simulink model "robust_simu"  (R2022a)
settings: Solver=VariableStepAuto  StartTime=0.0  StopTime=600  RelTol=1e-3
values from neighbouring files (symbols this model uses):
  ctrK_A = K.A    [robust.m]
  ctrK_B = K.B    [robust.m]
  ctrK_C = K.C    [robust.m]
  ctrK_D = K.D    [robust.m]
  ctrKpre_A = K_pre.A    [robust.m]
  ctrKpre_B = K_pre.B    [robust.m]
  ctrKpre_C = K_pre.C    [robust.m]
  ctrKpre_D = K_pre.D    [robust.m]
  G_A = sys_G.A    [robust.m]
  G_B = sys_G.B    [robust.m]
  G_C = sys_G.C    [robust.m]
  G_D = sys_G.D    [robust.m]
  Gd_A = sys_Gd.A    [robust.m]
  Gd_B = sys_Gd.B    [robust.m]
  Gd_C = sys_Gd.C    [robust.m]
  Gd_D = sys_Gd.D    [robust.m]
settings Model: Creator=Linxi Ren  LastModifiedBy=Linxi Ren

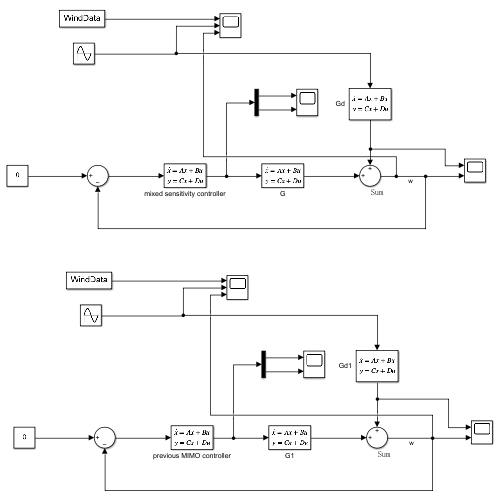
[thumbnail: Simulink's stored preview of the top-level diagram]
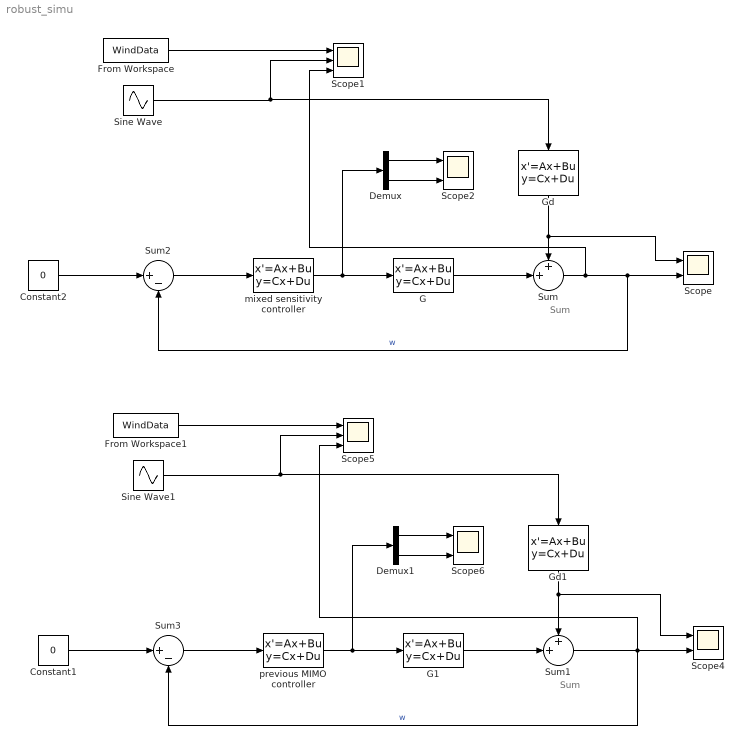
== system robust_simu ==
  note: Sum
  note: Sum
  Constant1 : Constant  Value=0
  Constant2 : Constant  Value=0
  Demux : Demux  Outputs=2
  Demux1 : Demux  Outputs=2
  From Workspace : FromWorkspace  VariableName=WindData  SampleTime=0.01
  From Workspace1 : FromWorkspace  VariableName=WindData  SampleTime=0.01
  G : StateSpace  A=G_A  B=G_B  C=G_C  D=G_D  InitialCondition=0
  G1 : StateSpace  A=G_A  B=G_B  C=G_C  D=G_D  InitialCondition=0
  Gd : StateSpace  A=Gd_A  B=Gd_B  C=Gd_C  D=Gd_D  InitialCondition=0
  Gd1 : StateSpace  A=Gd_A  B=Gd_B  C=Gd_C  D=Gd_D  InitialCondition=0
  Scope{,2,4,6} (4 alike) : Scope  NumInputPorts=2
  Scope1 : Scope  NumInputPorts=3
  Scope5 : Scope  NumInputPorts=3
  Sine Wave : Sin  Amplitude=2  Frequency=0.002*pi  SampleTime=0
  Sine Wave1 : Sin  Amplitude=2  Frequency=0.002*pi  SampleTime=0
  Sum : Sum  Inputs=++|
  Sum1 : Sum  Inputs=++|
  Sum2 : Sum  Inputs=|+-
  Sum3 : Sum  Inputs=|+-
  mixed sensitivity controller : StateSpace  A=ctrK_A  B=ctrK_B  C=ctrK_C  D=ctrK_D  InitialCondition=0
  previous MIMO controller : StateSpace  A=ctrKpre_A  B=ctrKpre_B  C=ctrKpre_C  D=ctrKpre_D  InitialCondition=0
  wires:
  Sine Wave/1 -> Gd/1, Scope1/2
  G/1 -> Sum/2
  Gd/1 -> Scope/1, Sum/1
  Sum2/1 -> mixed sensitivity controller/1
  Sum/1 -> Scope1/3, Scope/2, Sum2/2  "w"
  Demux/2 -> Scope2/2
  Demux/1 -> Scope2/1
  From Workspace/1 -> Scope1/1
  Constant2/1 -> Sum2/1
  mixed sensitivity controller/1 -> Demux/1, G/1
  Sum1/1 -> Scope5/3, Scope4/2, Sum3/2  "w"
  Demux1/2 -> Scope6/2
  Demux1/1 -> Scope6/1
  Gd1/1 -> Scope4/1, Sum1/1
  G1/1 -> Sum1/2
  Sine Wave1/1 -> Gd1/1, Scope5/2
  Sum3/1 -> previous MIMO controller/1
  previous MIMO controller/1 -> Demux1/1, G1/1
  From Workspace1/1 -> Scope5/1
  Constant1/1 -> Sum3/1
